simulink model "AircraftSimulink_2"  (R2020b)
settings: Solver=VariableStepAuto  StartTime=0.0  StopTime=T  RelTol=1e-3
values from neighbouring files (symbols this model uses):
  P = [20.4 ... (first row only)    [IntialConditions.m]
  U = [24.1371 ... (first row only)    [IntialConditions.m]    (also in cost_lvl_flight.m = Z(10:15))
  Xi = [79.9177 ... (first row only)    [IntialConditions.m]
undefined symbols (not defined in the file or in its folder): AircraftModel, NAV
libraries: aerolibutil x2, sharedutil x1, vrlib x1
settings Model: Creator=HP  LastModifiedBy=HP

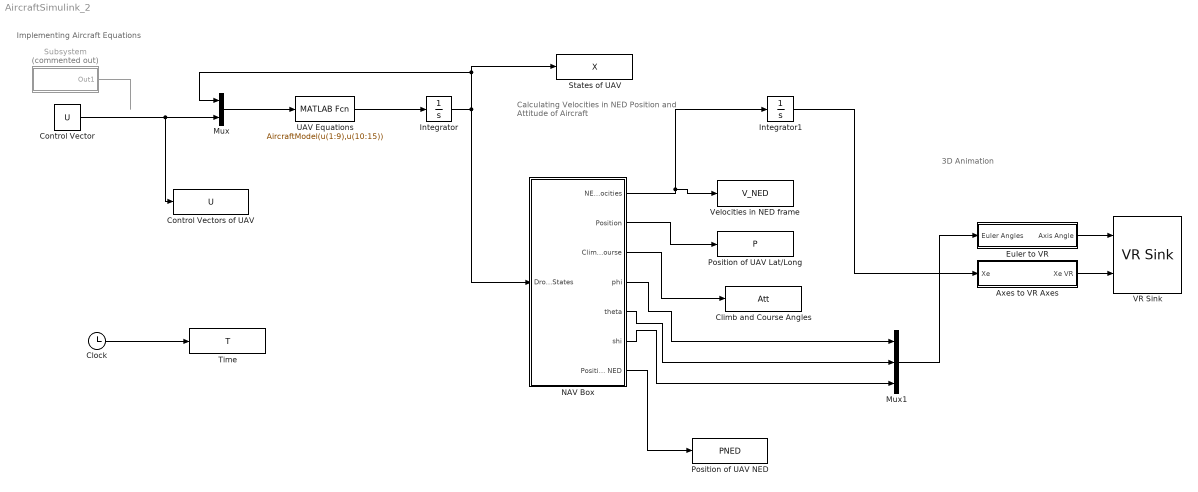
== system AircraftSimulink_2 ==
  note: Calculating Velocities in NED
      | Position and Attitude of
      | Aircraft
  note: Implementing Aircraft Equations
  note: 3D Animation
  Axes to VR Axes : Subsystem
  Climb and Course Angles : ToWorkspace  VariableName=Att  SampleTime=-1
  Clock : Clock
  Control Vector : Constant  Value=U
  Control Vectors of UAV : ToWorkspace  VariableName=U  SampleTime=-1
  Euler to VR : Subsystem
  Integrator : Integrator  InitialCondition=Xi
  Integrator1 : Integrator
  Mux : Mux  Inputs=2
  Mux1 : Mux  Inputs=3
  NAV Box : Subsystem
  Position of UAV Lat/Long : ToWorkspace  VariableName=P  SampleTime=-1
  Position of UAV NED : ToWorkspace  VariableName=PNED  SampleTime=-1
  States of UAV : ToWorkspace  VariableName=X  SampleTime=-1
  Subsystem : Subsystem  Commented=on
  Time : ToWorkspace  VariableName=T  SampleTime=-1
  UAV Equations : MATLABFcn  MATLABFcn=AircraftModel(u(1:9),u(10:15))
  VR Sink : vrlib/VR Sink  InstantiateOnLoad=on  SampleTime=0.1  ViewEnable=on  RemoteChange=off  RemoteView=off  FieldsWritten=HL20.rotation.4.1.1.double#HL20.translation.3.1.1.double  WorldFileName=aeroblk_HL20.wrl  WorldDescription=aeroblk_HL20  AutoView=on  VideoDimensions=[]  AllowVariableSize=off  FigureProperties="{'Position', 'Name', 'Viewpoint', 'CameraBound', 'CameraDirection', 'CameraPosition', 'CameraUpVector', 'ZoomFactor', 'Antialiasing', 'Headlight', 'Lighting', 'NavPanel', 'Sound', 'StatusBar', 'Stereo3D', 'Stereo3DCameraOffset', 'Stereo3DHIT', 'ToolBar', 'Textures', 'Transparency', 'Triad', 'Wireframe', 'NavZones', 'NavMode', 'NavSpeed', 'CaptureFileFormat', 'CaptureFileName', 'Record2DCompressMethod', 'Record2DCompressQuality', 'Record2D', 'Record2DFileName', 'Record2DFPS'; [1.0000000000000000e+00   7.4199999999999932e+01   1.5360000000000000e+03   7.3880000000000007e+02], 'aeroblk_HL20', 'Rear Position', 'on', [0.0000000000000000e+00   0.0000000000000000e+00  -1.0000000000000000e+00], [0.0000000000000000e+00   0.0000000000000000e+00   0.0000000000000000e+00], [0.0000000000000000e+00   1.0000000000000000e+00   0.0000000000000000e+00], [1.0000000000000000e+00], 'on', 'on', 'on', 'halfbar', 'on', 'on', 'off', [1.0000000149011612e-01], [0.0000000000000000e+00], 'on', 'on', 'on', 'none', 'off', 'off', 'fly', 'normal', 'tif', '%f_anim_%n.tif', 'auto', [7.5000000000000000e+01], 'off', '%f_anim_%n.avi', 'auto'}"
  Velocities in NED frame : ToWorkspace  VariableName=V_NED  SampleTime=-1
  wires:
  Integrator/1 -> NAV Box/1(Drone States), States of UAV/1, Mux/1
  UAV Equations/1 -> Integrator/1
  Clock/1 -> Time/1
  NAV Box/2(Position) -> Position of UAV Lat/Long/1
  NAV Box/3(Climb and Course) -> Climb and Course Angles/1
  NAV Box/1(NED Velocities) -> Integrator1/1, Velocities in NED frame/1
  Axes to VR Axes/1(Xe VR) -> VR Sink/2
  Euler to VR/1(Axis Angle) -> VR Sink/1
  Mux1/1 -> Euler to VR/1(Euler Angles)
  NAV Box/4(phi) -> Mux1/1
  NAV Box/5(theta) -> Mux1/2
  NAV Box/6(shi) -> Mux1/3
  Integrator1/1 -> Axes to VR Axes/1(Xe)
  NAV Box/7(Position NED) -> Position of UAV NED/1
  Mux/1 -> UAV Equations/1
  Subsystem/1(Out1) -> ?
  Control Vector/1 -> Control Vectors of UAV/1, Mux/2

== system AircraftSimulink_2/Axes to VR Axes ==
  Xe : Inport
  Concatenate : Concatenate  NumInputs=3
  Demux : Demux  Outputs=3
      settings: DisplayOption=none
  rad-->deg : Gain  Gain=-1  SaturateOnIntegerOverflow=on  OutDataTypeStr=Inherit: Same as input  ParamDataTypeStr=Inherit: Same as input
  rad-->deg1 : Gain  Gain=-1  SaturateOnIntegerOverflow=on  OutDataTypeStr=Inherit: Same as input  ParamDataTypeStr=Inherit: Same as input
  Xe VR : Outport  VectorParamsAs1DForOutWhenUnconnected=off
  wires:
  Xe/1 -> Demux/1
  Demux/1 -> Concatenate/1
  Demux/2 -> rad-->deg/1
  Demux/3 -> rad-->deg1/1
  Concatenate/1 -> Xe VR/1
  rad-->deg1/1 -> Concatenate/2
  rad-->deg/1 -> Concatenate/3

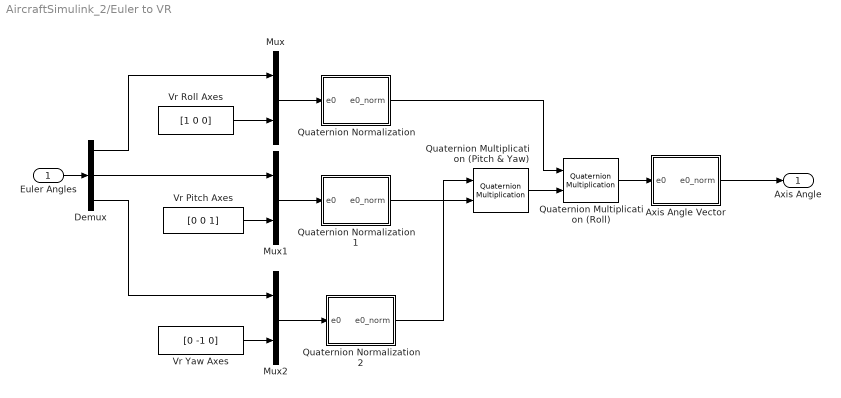
== system AircraftSimulink_2/Euler to VR ==
  Euler Angles : Inport
  Axis Angle Vector : Subsystem
  Demux : Demux  Outputs=3
      settings: DisplayOption=none
  Mux : Mux  Inputs=2
  Mux1 : Mux  Inputs=2
  Mux2 : Mux  Inputs=2
  Quaternion Multiplication (Pitch & Yaw) : aerolibutil/Quaternion Multiplication
  Quaternion Multiplication (Roll) : aerolibutil/Quaternion Multiplication
  Quaternion Normalization : Subsystem
  Quaternion Normalization1 : Subsystem
  Quaternion Normalization2 : Subsystem
  Vr Pitch Axes : Constant  Value=[0 0 1]
  Vr Roll Axes : Constant  Value=[1 0 0]
  Vr Yaw Axes : Constant  Value=[0 -1 0]
  Axis Angle : Outport  VectorParamsAs1DForOutWhenUnconnected=off
  wires:
  Quaternion Multiplication (Roll)/1 -> Axis Angle Vector/1(e0)
  Quaternion Multiplication (Pitch & Yaw)/1 -> Quaternion Multiplication (Roll)/2
  Axis Angle Vector/1(e0_norm) -> Axis Angle/1
  Quaternion Normalization/1(e0_norm) -> Quaternion Multiplication (Roll)/1
  Quaternion Normalization2/1(e0_norm) -> Quaternion Multiplication (Pitch & Yaw)/1
  Quaternion Normalization1/1(e0_norm) -> Quaternion Multiplication (Pitch & Yaw)/2
  Mux2/1 -> Quaternion Normalization2/1(e0)
  Mux1/1 -> Quaternion Normalization1/1(e0)
  Mux/1 -> Quaternion Normalization/1(e0)
  Demux/3 -> Mux2/1
  Vr Yaw Axes/1 -> Mux2/2
  Demux/2 -> Mux1/1
  Vr Pitch Axes/1 -> Mux1/2
  Demux/1 -> Mux/1
  Vr Roll Axes/1 -> Mux/2
  Euler Angles/1 -> Demux/1

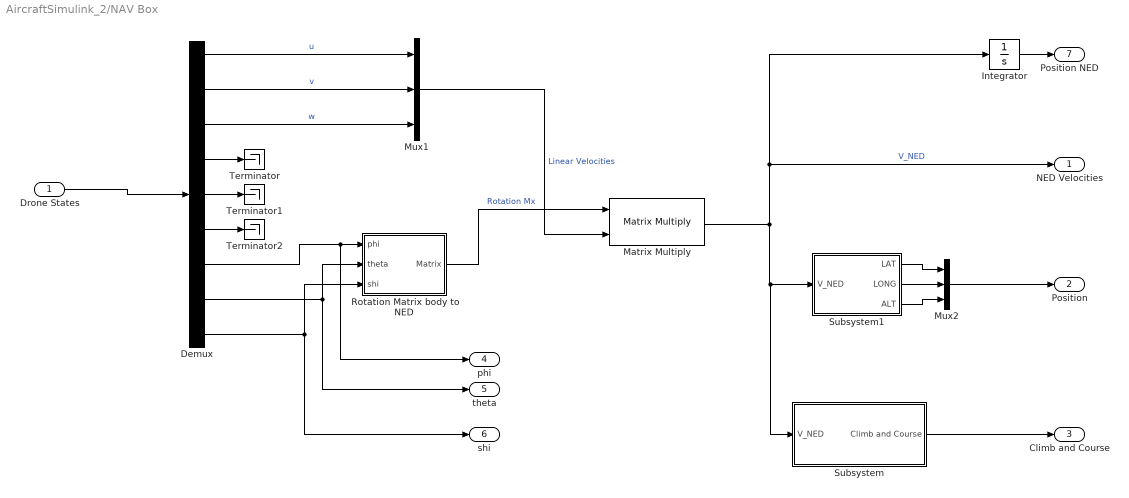
== system AircraftSimulink_2/NAV Box ==
  Drone States : Inport
  Demux : Demux  Outputs=9
  Integrator : Integrator
  Matrix Multiply : Product  Multiplication=Matrix(*)
  Mux1 : Mux  Inputs=3
  Mux2 : Mux  Inputs=3
  Rotation Matrix body to NED : Subsystem
  Subsystem : Subsystem
  Subsystem1 : Subsystem
  Terminator : Terminator
  Terminator1 : Terminator
  Terminator2 : Terminator
  NED Velocities : Outport
  Position : Outport  Port=2
  Climb and Course : Outport  Port=3
  phi : Outport  Port=4
  theta : Outport  Port=5
  shi : Outport  Port=6
  Position NED : Outport  Port=7
  wires:
  Subsystem1/1(LAT) -> Mux2/1
  Matrix Multiply/1 -> Integrator/1, NED Velocities/1, Subsystem/1("V_NED "), Subsystem1/1(V_NED)  "V_NED"
  Subsystem1/3(ALT) -> Mux2/3
  Subsystem1/2(LONG) -> Mux2/2
  Rotation Matrix body to NED/1(Matrix) -> Matrix Multiply/1  "Rotation Mx"
  Mux1/1 -> Matrix Multiply/2  "Linear Velocities"
  Demux/7 -> phi/1, Rotation Matrix body to NED/1(phi)
  Demux/9 -> Rotation Matrix body to NED/3(shi), shi/1
  Demux/6 -> Terminator2/1
  Demux/2 -> Mux1/2  "v"
  Demux/8 -> Rotation Matrix body to NED/2(theta), theta/1
  Demux/1 -> Mux1/1  "u"
  Demux/3 -> Mux1/3  "w"
  Drone States/1 -> Demux/1
  Mux2/1 -> Position/1
  Demux/5 -> Terminator1/1
  Demux/4 -> Terminator/1
  Subsystem/1(Climb and Course) -> Climb and Course/1
  Integrator/1 -> Position NED/1

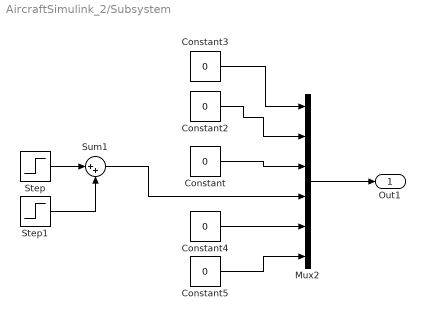
== system AircraftSimulink_2/Subsystem ==
  Constant{,2..5} (5 alike) : Constant  Value=0
  Mux2 : Mux  Inputs=6
  Step : Step  Time=10  After=-5  SampleTime=0
  Step1 : Step  Time=15  After=5  SampleTime=0
  Sum1 : Sum  Inputs=|++
  Out1 : Outport
  wires:
  Mux2/1 -> Out1/1
  Constant2/1 -> Mux2/2
  Constant3/1 -> Mux2/1
  Constant4/1 -> Mux2/5
  Step/1 -> Sum1/1
  Constant5/1 -> Mux2/6
  Step1/1 -> Sum1/2
  Sum1/1 -> Mux2/4
  Constant/1 -> Mux2/3

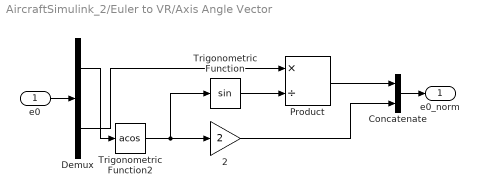
== system AircraftSimulink_2/Euler to VR/Axis Angle Vector ==
  e0 : Inport
  2 : Gain  Gain=2  SaturateOnIntegerOverflow=on  OutDataTypeStr=Inherit: Same as input  ParamDataTypeStr=Inherit: Same as input
  Concatenate : Concatenate
  Demux : Demux  Outputs=[1 3 ]
      settings: DisplayOption=none
  Product : Product  Inputs=*/  InputSameDT=on  SaturateOnIntegerOverflow=on  OutDataTypeStr=Inherit: Same as first input
  Trigonometric Function : Trigonometry
  Trigonometric Function2 : Trigonometry  Operator=acos
  e0_norm : Outport  VectorParamsAs1DForOutWhenUnconnected=off
  wires:
  Demux/1 -> Trigonometric Function2/1
  Demux/2 -> Product/1
  Concatenate/1 -> e0_norm/1
  Product/1 -> Concatenate/1
  2/1 -> Concatenate/2
  Trigonometric Function/1 -> Product/2
  Trigonometric Function2/1 -> Trigonometric Function/1, 2/1
  e0/1 -> Demux/1

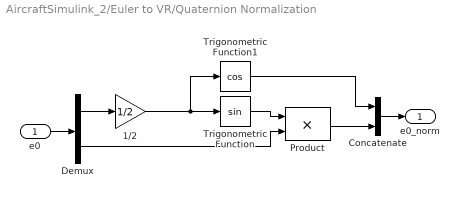
== system AircraftSimulink_2/Euler to VR/Quaternion Normalization ==
  e0 : Inport
  1/2 : Gain  Gain=1/2  SaturateOnIntegerOverflow=on  OutDataTypeStr=Inherit: Same as input  ParamDataTypeStr=Inherit: Same as input
  Concatenate : Concatenate
  Demux : Demux  Outputs=[1 3]
      settings: DisplayOption=none
  Product : Product  InputSameDT=on  SaturateOnIntegerOverflow=on  OutDataTypeStr=Inherit: Same as first input
  Trigonometric Function : Trigonometry
  Trigonometric Function1 : Trigonometry  Operator=cos
  e0_norm : Outport  VectorParamsAs1DForOutWhenUnconnected=off
  wires:
  Trigonometric Function1/1 -> Concatenate/1
  Demux/2 -> Product/2
  Demux/1 -> 1/2/1
  Concatenate/1 -> e0_norm/1
  Product/1 -> Concatenate/2
  Trigonometric Function/1 -> Product/1
  1/2/1 -> Trigonometric Function1/1, Trigonometric Function/1
  e0/1 -> Demux/1

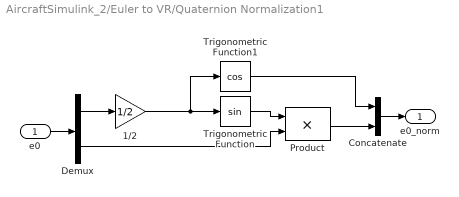
== system AircraftSimulink_2/Euler to VR/Quaternion Normalization1 ==
  e0 : Inport
  1/2 : Gain  Gain=1/2  SaturateOnIntegerOverflow=on  OutDataTypeStr=Inherit: Same as input  ParamDataTypeStr=Inherit: Same as input
  Concatenate : Concatenate
  Demux : Demux  Outputs=[1 3]
      settings: DisplayOption=none
  Product : Product  InputSameDT=on  SaturateOnIntegerOverflow=on  OutDataTypeStr=Inherit: Same as first input
  Trigonometric Function : Trigonometry
  Trigonometric Function1 : Trigonometry  Operator=cos
  e0_norm : Outport  VectorParamsAs1DForOutWhenUnconnected=off
  wires:
  e0/1 -> Demux/1
  1/2/1 -> Trigonometric Function/1, Trigonometric Function1/1
  Trigonometric Function/1 -> Product/1
  Product/1 -> Concatenate/2
  Concatenate/1 -> e0_norm/1
  Demux/1 -> 1/2/1
  Demux/2 -> Product/2
  Trigonometric Function1/1 -> Concatenate/1

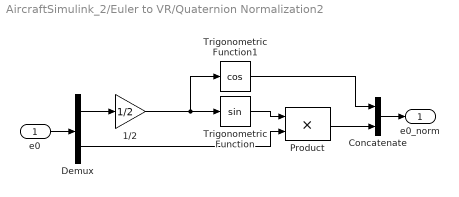
== system AircraftSimulink_2/Euler to VR/Quaternion Normalization2 ==
  e0 : Inport
  1/2 : Gain  Gain=1/2  SaturateOnIntegerOverflow=on  OutDataTypeStr=Inherit: Same as input  ParamDataTypeStr=Inherit: Same as input
  Concatenate : Concatenate
  Demux : Demux  Outputs=[1 3]
      settings: DisplayOption=none
  Product : Product  InputSameDT=on  SaturateOnIntegerOverflow=on  OutDataTypeStr=Inherit: Same as first input
  Trigonometric Function : Trigonometry
  Trigonometric Function1 : Trigonometry  Operator=cos
  e0_norm : Outport  VectorParamsAs1DForOutWhenUnconnected=off
  wires:
  Trigonometric Function1/1 -> Concatenate/1
  Demux/2 -> Product/2
  Demux/1 -> 1/2/1
  Concatenate/1 -> e0_norm/1
  Product/1 -> Concatenate/2
  Trigonometric Function/1 -> Product/1
  1/2/1 -> Trigonometric Function1/1, Trigonometric Function/1
  e0/1 -> Demux/1

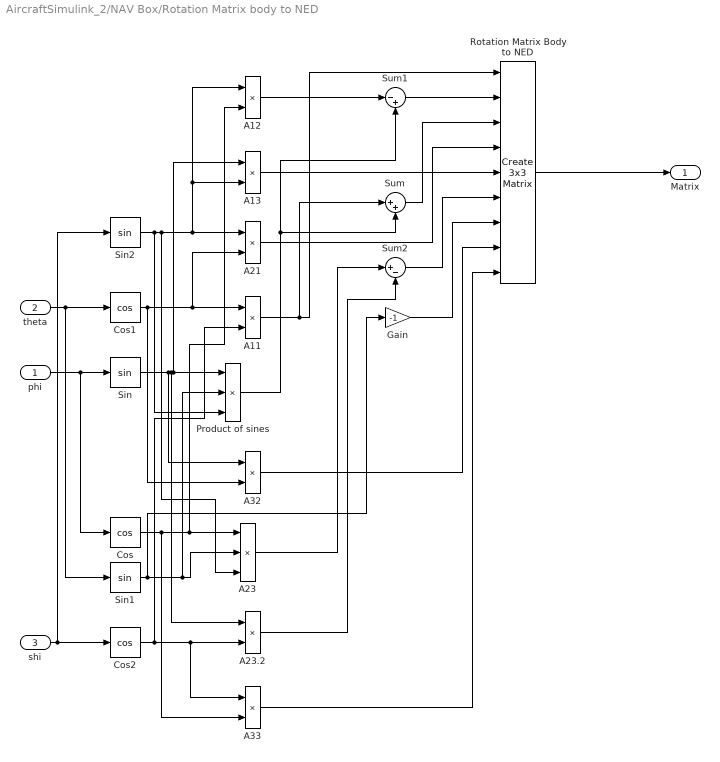
== system AircraftSimulink_2/NAV Box/Rotation Matrix body to NED ==
  phi : Inport
  theta : Inport  Port=2
  shi : Inport  Port=3
  A{11..13,21,32..33} (6 alike) : Product
  A23 : Product  Inputs=3
  A23.2 : Product
  Cos : Trigonometry  Operator=cos
  Cos1 : Trigonometry  Operator=cos
  Cos2 : Trigonometry  Operator=cos
  Gain : Gain  Gain=-1
  Product of sines : Product  Inputs=3
  Rotation Matrix Body to NED : sharedutil/Create 3x3 Matrix  aMode=aMode
      settings: SourceProductBaseCode=AE,PW,MT,UV,VE,VP
  Sin : Trigonometry
  Sin1 : Trigonometry
  Sin2 : Trigonometry
  Sum : Sum  Inputs=|++
  Sum1 : Sum  Inputs=|-+
  Sum2 : Sum  Inputs=|+-
  Matrix : Outport
  wires:
  A12/1 -> Sum1/1
  Rotation Matrix Body to NED/1 -> Matrix/1
  Sum1/1 -> Rotation Matrix Body to NED/2
  A33/1 -> Rotation Matrix Body to NED/9
  A23.2/1 -> Sum2/2
  Gain/1 -> Rotation Matrix Body to NED/7
  A11/1 -> Sum/1, Rotation Matrix Body to NED/1
  theta/1 -> Cos1/1, Sin1/1
  A21/1 -> Rotation Matrix Body to NED/4
  Sum/1 -> Rotation Matrix Body to NED/5
  A23/1 -> Sum2/1
  phi/1 -> Cos/1, Sin/1
  Sum2/1 -> Rotation Matrix Body to NED/6
  Cos2/1 -> A33/1, A23.2/2, A11/2
  A13/1 -> Rotation Matrix Body to NED/3
  Cos1/1 -> A21/2, A11/1, A32/2
  A32/1 -> Rotation Matrix Body to NED/8
  Product of sines/1 -> Sum/2, Sum1/2
  Sin1/1 -> Product of sines/2, A23/2, Gain/1
  shi/1 -> Cos2/1, Sin2/1
  Cos/1 -> A23/1, A12/2, A33/2
  Sin/1 -> Product of sines/1, A13/1, A23.2/1, A32/1
  Sin2/1 -> A13/2, A12/1, A21/1, A23/3, Product of sines/3

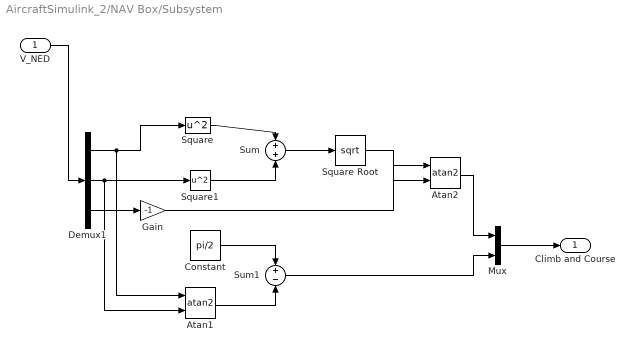
== system AircraftSimulink_2/NAV Box/Subsystem ==
  "V_NED " : Inport
  Atan1 : Trigonometry  Operator=atan2
  Atan2 : Trigonometry  Operator=atan2
  Constant : Constant  Value=pi/2
  Demux1 : Demux  Outputs=3
  Gain : Gain  Gain=-1
  Mux : Mux  Inputs=2
  Square : Math  Operator=square  SaturateOnIntegerOverflow=on
  Square Root : Sqrt  SaturateOnIntegerOverflow=on
  Square1 : Math  Operator=square  SaturateOnIntegerOverflow=on
  Sum : Sum  Inputs=+|+
  Sum1 : Sum  Inputs=+|-
  Climb and Course : Outport
  wires:
  Demux1/1 -> Square/1, Atan1/1
  Sum/1 -> Square Root/1
  Sum1/1 -> Mux/2
  Demux1/2 -> Square1/1, Atan1/2
  Gain/1 -> Atan2/1
  Square1/1 -> Sum/2
  Atan2/1 -> Mux/1
  Mux/1 -> Climb and Course/1
  Atan1/1 -> Sum1/2
  Square Root/1 -> Atan2/2
  Demux1/3 -> Gain/1
  Constant/1 -> Sum1/1
  Square/1 -> Sum/1
  "V_NED "/1 -> Demux1/1

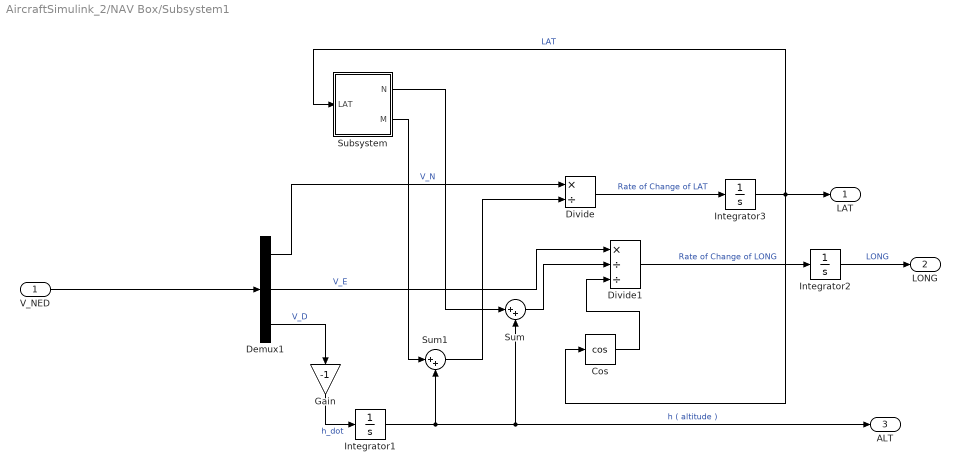
== system AircraftSimulink_2/NAV Box/Subsystem1 ==
  V_NED : Inport
  Cos : Trigonometry  Operator=cos
  Demux1 : Demux  Outputs=3
  Divide : Product  Inputs=*/
  Divide1 : Product  Inputs=*//
  Gain : Gain  Gain=-1
  Integrator1 : Integrator  InitialCondition=P(3)
  Integrator2 : Integrator  InitialCondition=P(2)
  Integrator3 : Integrator  InitialCondition=P(1)
  Subsystem : Subsystem
  Sum : Sum  Inputs=|++
  Sum1 : Sum  Inputs=|++
  LAT : Outport
  LONG : Outport  Port=2
  ALT : Outport  Port=3
  wires:
  Integrator1/1 -> ALT/1, Sum/2, Sum1/2  "h ( altitude )"
  Demux1/1 -> Divide/1  "V_N"
  Divide1/1 -> Integrator2/1  "Rate of Change of LONG"
  Gain/1 -> Integrator1/1  "h_dot"
  Sum1/1 -> Divide/2
  Demux1/3 -> Gain/1  "V_D"
  Divide/1 -> Integrator3/1  "Rate of Change of LAT"
  Demux1/2 -> Divide1/1  "V_E"
  Integrator3/1 -> Cos/1, Subsystem/1(LAT), LAT/1  "LAT"
  Sum/1 -> Divide1/2
  Subsystem/2(M) -> Sum1/1
  Subsystem/1(N) -> Sum/1
  V_NED/1 -> Demux1/1
  Integrator2/1 -> LONG/1  "LONG"
  Cos/1 -> Divide1/3

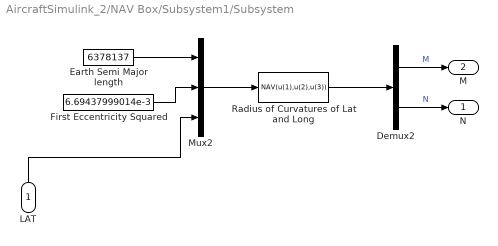
== system AircraftSimulink_2/NAV Box/Subsystem1/Subsystem ==
  LAT : Inport
  Demux2 : Demux  Outputs=2
  Earth Semi Major length : Constant  Value=6378137
  First Eccentricity Squared : Constant  Value=6.69437999014e-3
  Mux2 : Mux  Inputs=3
  Radius of Curvatures of Lat and Long : MATLABFcn  MATLABFcn=NAV(u(1),u(2),u(3))
  N : Outport
  M : Outport  Port=2
  wires:
  Demux2/1 -> M/1  "M"
  Earth Semi Major length/1 -> Mux2/1
  Demux2/2 -> N/1  "N"
  Mux2/1 -> Radius of Curvatures of Lat and Long/1
  Radius of Curvatures of Lat and Long/1 -> Demux2/1
  First Eccentricity Squared/1 -> Mux2/2
  LAT/1 -> Mux2/3
